simulink model "examples"  (R2023b)
settings: Solver=FixedStepDiscrete  StartTime=0.0  StopTime=10  FixedStep=0.1
values from neighbouring files (symbols this model uses):
  x = 120    [matlab.mat]
libraries: simulink x6
settings Model: Creator=DELL  LastModifiedBy=DELL
settings OptimizationCC: DefaultParameterBehavior=Inlined  UseDivisionForNetSlopeComputation=on  GainParamInheritBuiltInType=on  UseFloatMulNetSlope=on  InlineInvariantSignals=on  PassReuseOutputArgsAs=Individual arguments  ZeroExternalMemoryAtStartup=off  ZeroInternalMemoryAtStartup=off  NoFixptDivByZeroProtection=on  EfficientFloat2IntCast=on  LifeSpan=1  OptimizeBlockOrder=speed  DifferentSizesBufferReuse=on  EfficientTunableParamExpr=on
settings DebuggingCC: ParameterTunabilityLossMsg=error
settings HardwareCC: ProdBitPerPointer=32  ProdBitPerSizeT=32  ProdBitPerPtrDiffT=32  ProdLargestAtomicInteger=Long  ProdLargestAtomicFloat=Double  ProdWordSize=32  ProdLongLongMode=on  ProdHWDeviceType=ARM Compatible->ARM Cortex-M
settings SFSimCC: MATLABDynamicMemAlloc=off
settings RTWCC: Description=Embedded Coder  SystemTargetFile=ert.tlc  TemplateMakefile=ert_default_tmf
settings CodeAppCC: ForceParamTrailComments=on  IgnoreCustomStorageClasses=off  OperatorAnnotations=on  SimulinkDataObjDesc=on  SFDataObjDesc=on  CustomSymbolStrGlobalVar=rt$N$M  CustomSymbolStrType=$N$M  CustomSymbolStrFcn=$N$M$F  CustomSymbolStrMacro=$N$M  InsertBlockDesc=on
settings ERTTargetCC: TargetLangStandard=C99 (ISO)  GenerateSampleERTMain=on  IncludeMdlTerminateFcn=off  CombineSignalStateStructs=on  SuppressErrorStatus=on  SupportAbsoluteTime=off  SupportComplex=off  InlinedParameterPlacement=NonHierarchical  ERTCustomFileTemplate=example_file_process.tlc  ERTFilePackagingFormat=CompactWithDataFile

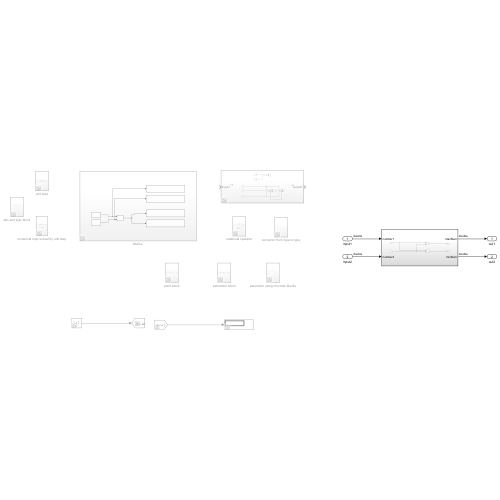
[thumbnail: Simulink's stored preview of the top-level diagram]
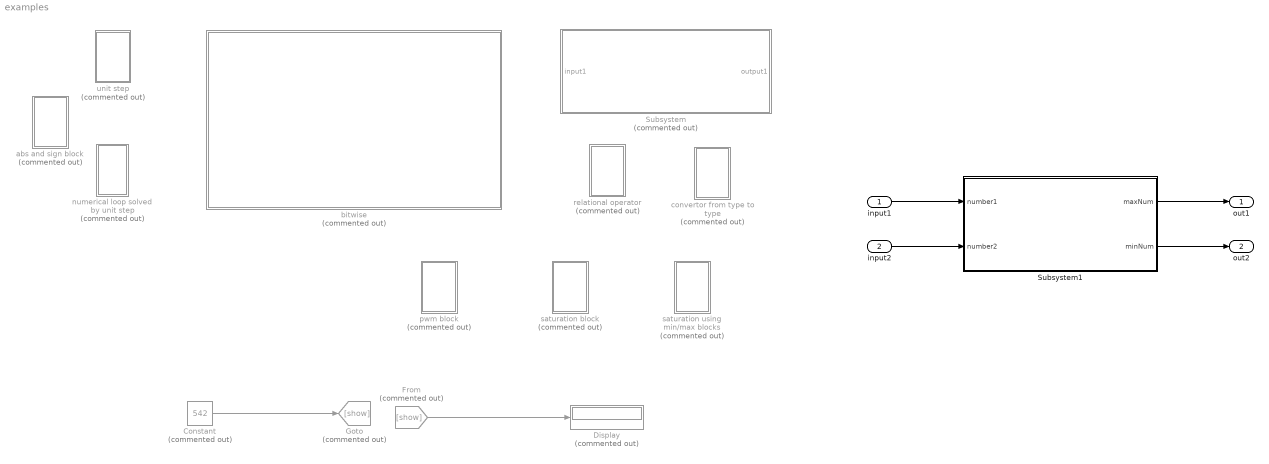
== system examples ==
  input1 : Inport
  input2 : Inport  Port=2
  Constant : Constant  Commented=on  Value=542
  Display : Display  Commented=on
  From : From  Commented=on  GotoTag=show
  Goto : Goto  Commented=on  GotoTag=show
  Subsystem : Subsystem  Commented=on
  Subsystem1 : Subsystem
  abs and sign block : Subsystem  Commented=on
  "bitwise " : Subsystem  Commented=on
  convertor from type to type : Subsystem  Commented=on
  numerical loop solved by unit step : Subsystem  Commented=on
  pwm block : Subsystem  Commented=on
  relational operator : Subsystem  Commented=on
  saturation block : Subsystem  Commented=on
  saturation using min/max blocks : Subsystem  Commented=on
  unit step : Subsystem  Commented=on
  out1 : Outport
  out2 : Outport  Port=2
  wires:
  Constant/1 -> Goto/1
  From/1 -> Display/1
  Subsystem1/1(maxNum) -> out1/1
  Subsystem1/2(minNum) -> out2/1
  input1/1 -> Subsystem1/1(number1)
  input2/1 -> Subsystem1/2(number2)

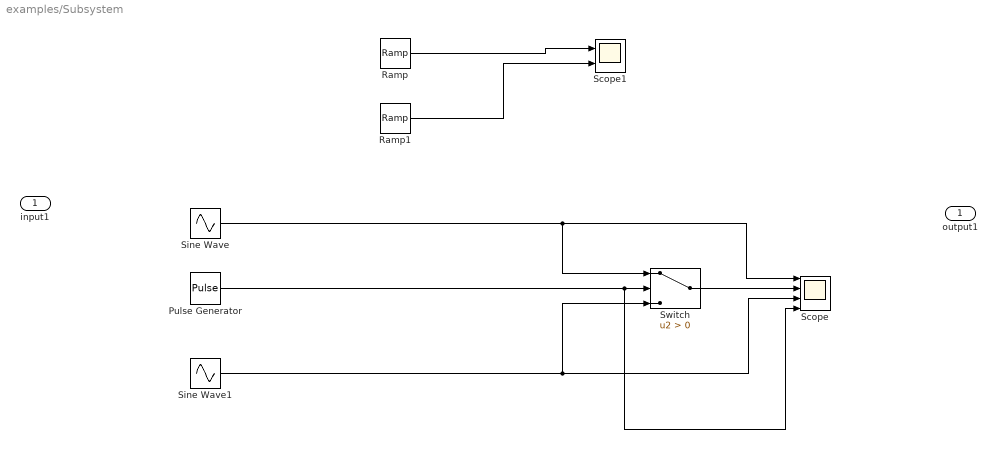
== system examples/Subsystem ==
  input1 : Inport
  Pulse Generator : DiscretePulseGenerator  PulseType=Time based  Period=10  PulseWidth=50
  Ramp : simulink/Sources/Ramp  slope=2  start=0  InitialOutput=5
  Ramp1 : simulink/Sources/Ramp  slope=-2  start=0  InitialOutput=5
  Scope : Scope  NumInputPorts=4
  Scope1 : Scope  NumInputPorts=2
  Sine Wave : Sin  SampleTime=0
  Sine Wave1 : Sin  Phase=-pi  SampleTime=0
  Switch : Switch  Criteria=u2 > Threshold  SaturateOnIntegerOverflow=off  InputSameDT=off
  output1 : Outport
  wires:
  Switch/1 -> Scope/2
  Sine Wave/1 -> Scope/1, Switch/1
  Ramp/1 -> Scope1/1
  Pulse Generator/1 -> Scope/4, Switch/2
  Sine Wave1/1 -> Switch/3, Scope/3
  Ramp1/1 -> Scope1/2

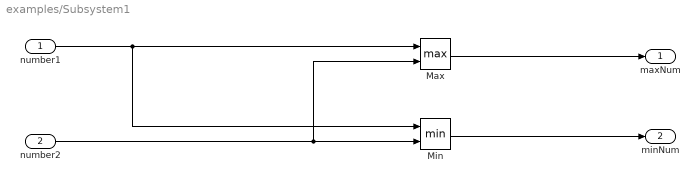
== system examples/Subsystem1 ==
  number1 : Inport
  number2 : Inport  Port=2
  Max : MinMax  Function=max  Inputs=2
  Min : MinMax  Inputs=2
  maxNum : Outport
  minNum : Outport  Port=2
  wires:
  number2/1 -> Max/2, Min/2
  number1/1 -> Max/1, Min/1
  Min/1 -> minNum/1
  Max/1 -> maxNum/1

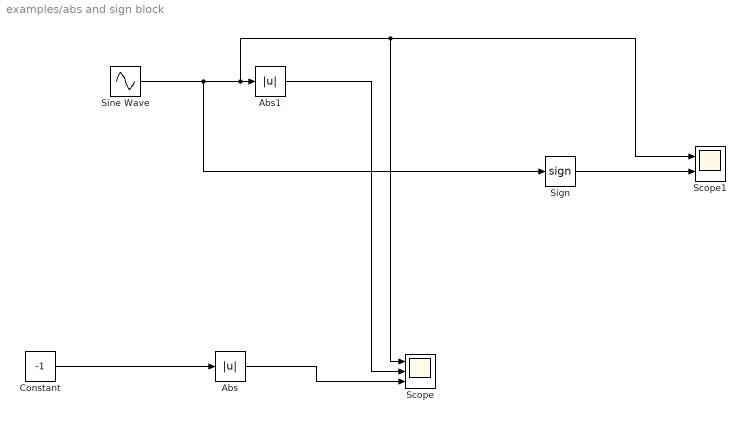
== system examples/abs and sign block ==
  Abs : Abs  RndMeth=Zero  SaturateOnIntegerOverflow=off
  Abs1 : Abs  ZeroCross=off  RndMeth=Zero
      settings: LockScale=on
  Constant : Constant  Value=-1
  Scope : Scope  NumInputPorts=3
  Scope1 : Scope  NumInputPorts=2
  Sign : Signum
  Sine Wave : Sin  SampleTime=0
  wires:
  Abs/1 -> Scope/3
  Sine Wave/1 -> Sign/1, Scope/1, Scope1/1, Abs1/1
  Sign/1 -> Scope1/2
  Constant/1 -> Abs/1
  Abs1/1 -> Scope/2

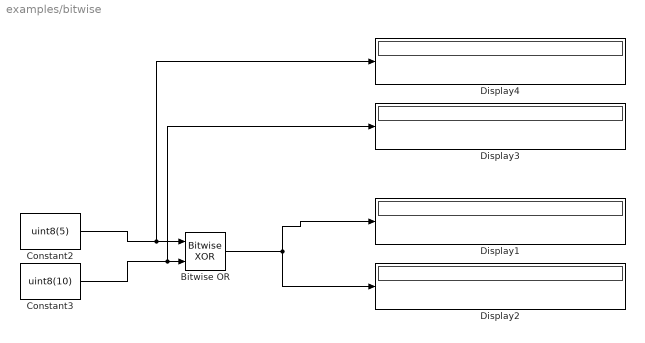
== system examples/bitwise  ==
  Bitwise OR : simulink/Logic and Bit Operations/Bitwise Operator  logicop=XOR  UseBitMask=off  NumInputPorts=2  BitMask=bin2dec('11011001')  BitMaskRealWorld=Stored Integer
      settings: LibrarySourceBlock=|
      | simulink/Quick Insert/Logic and Bit
      | Operations/Bitwise OR
  Constant2 : Constant  Value=uint8(5)
  Constant3 : Constant  Value=uint8(10)
  Display{1..4} (4 alike) : Display
      Display1 settings: Format=binary (Stored Integer)
      Display3 settings: Format=binary (Stored Integer)
      Display4 settings: Format=binary (Stored Integer)
  wires:
  Bitwise OR/1 -> Display1/1, Display2/1
  Constant3/1 -> Display3/1, Bitwise OR/2
  Constant2/1 -> Display4/1, Bitwise OR/1

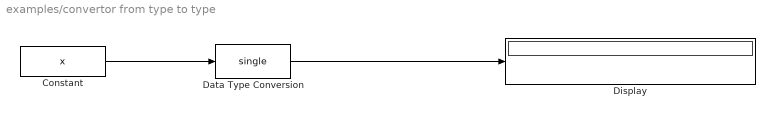
== system examples/convertor from type to type ==
  Constant : Constant  Value=x
  Data Type Conversion : DataTypeConversion  OutDataTypeStr=single  RndMeth=Round  SaturateOnIntegerOverflow=off
  Display : Display
  wires:
  Constant/1 -> Data Type Conversion/1
  Data Type Conversion/1 -> Display/1

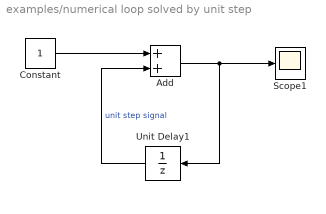
== system examples/numerical loop solved by unit step ==
  Add : Sum
  Constant : Constant
  Scope1 : Scope
  Unit Delay1 : UnitDelay  SampleTime=-1  HasFrameUpgradeWarning=on
  wires:
  Unit Delay1/1 -> Add/2  "unit step signal"
  Constant/1 -> Add/1
  Add/1 -> Unit Delay1/1, Scope1/1

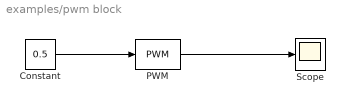
== system examples/pwm block ==
  Constant : Constant  Value=0.5
  PWM : simulink/Discontinuities/PWM  DisableCoverage=on  Period=2  InitialDelay=0  DisallowZeroDutyCycle=off  RunAtFixedTimeIntervals=off  SampleTime=0.1
  Scope : Scope
  wires:
  Constant/1 -> PWM/1
  PWM/1 -> Scope/1

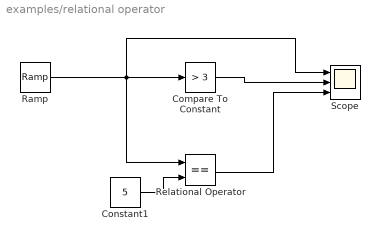
== system examples/relational operator ==
  Compare To Constant : simulink/Logic and Bit Operations/Compare To Constant  relop=>  const=3  OutDataTypeStr=boolean
  Constant1 : Constant  Value=5
  Ramp : simulink/Sources/Ramp  slope=1  start=0  InitialOutput=-0.5
  Relational Operator : RelationalOperator  Operator===  OutDataTypeStr=boolean  RndMeth=Simplest  InputSameDT=off
  Scope : Scope  NumInputPorts=3
  wires:
  Compare To Constant/1 -> Scope/2
  Ramp/1 -> Relational Operator/1, Scope/1, Compare To Constant/1
  Constant1/1 -> Relational Operator/2
  Relational Operator/1 -> Scope/3

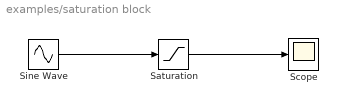
== system examples/saturation block ==
  Saturation : Saturate
  Scope : Scope
  Sine Wave : Sin  SampleTime=0
  wires:
  Saturation/1 -> Scope/1
  Sine Wave/1 -> Saturation/1

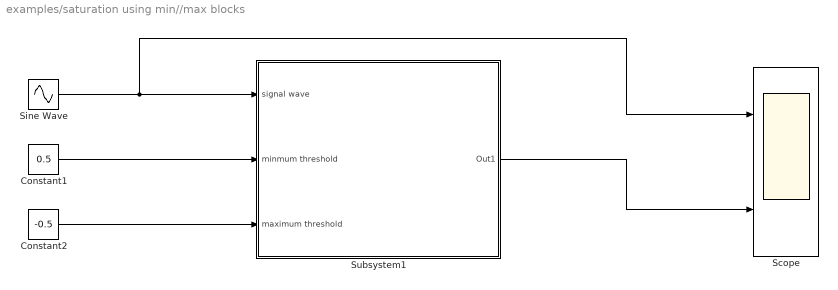
== system examples/saturation using min//max blocks ==
  Constant1 : Constant  Value=0.5
  Constant2 : Constant  Value=-0.5
  Scope : Scope  NumInputPorts=2
  Sine Wave : Sin  SampleTime=0
  Subsystem1 : Subsystem
  wires:
  Sine Wave/1 -> Scope/1, Subsystem1/1(signal wave)
  Constant2/1 -> Subsystem1/3(maximum threshold)
  Subsystem1/1(Out1) -> Scope/2
  Constant1/1 -> Subsystem1/2(minmum threshold)

== system examples/unit step ==
  Pulse Generator : DiscretePulseGenerator  PulseType=Time based  Period=1  PulseWidth=50
  Scope : Scope  NumInputPorts=2
  Unit Delay : UnitDelay  SampleTime=-1  HasFrameUpgradeWarning=on
  wires:
  Pulse Generator/1 -> Scope/1, Unit Delay/1  "original signal"
  Unit Delay/1 -> Scope/2  "unit step signal"

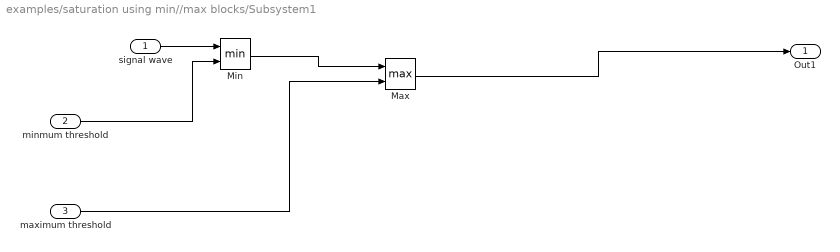
== system examples/saturation using min//max blocks/Subsystem1 ==
  signal wave : Inport
  minmum threshold : Inport  Port=2
  maximum threshold : Inport  Port=3
  Max : MinMax  Function=max  Inputs=2
  Min : MinMax  Inputs=2
  Out1 : Outport
  wires:
  Min/1 -> Max/1
  minmum threshold/1 -> Min/2
  Max/1 -> Out1/1
  maximum threshold/1 -> Max/2
  signal wave/1 -> Min/1
